simulink model "EE463_SoftwareProject2_q2_DCMotorDrive"  (R2017b)
settings: Solver=VariableStepDiscrete  StartTime=0.0  StopTime=2  RelTol=1e-3
libraries: powerlib x10
settings Model: Creator=mertelmas  LastModifiedBy=SiF

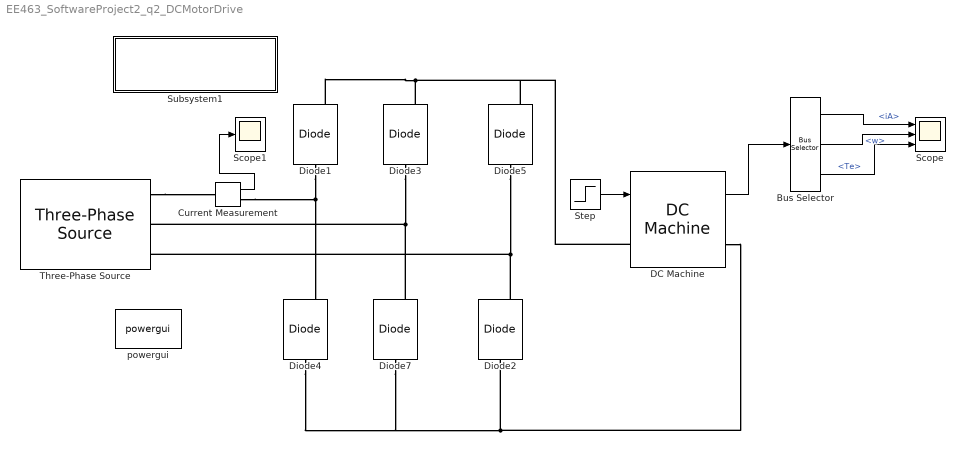
== system EE463_SoftwareProject2_q2_DCMotorDrive ==
  Bus Selector : BusSelector  OutputSignals=iA,w,Te
  Current Measurement : powerlib/Measurements/Current Measurement  PhasorSimulation=off  OutputType=Complex  PSBequivalent=0
  DC Machine : powerlib/Machines/DC Machine  PresetModel=No  MechanicalLoad=Torque TL  FieldType=Permanent magnet  ShowDetailedParameters=on  MeasurementBus=on  RLa="[ 10  0.01]"  RLf="[ 240  120]"  Laf=1.8  MachineConstant=Back-emf constant (V/rpm)  Ke=0.3  Kt=1.8  J=0.4  Bm=0  Tf=0  w0=0  Ifinit=0  TsPowergui=0  TsBlock=-1
  Diode{1..5,7} (6 alike) : powerlib/Power Electronics/Diode  Ron=0.001  Lon=0  Vf=0.8  IC=0  UseSnubber=0  Rs=500  Cs=250e-9  Measurements=on
  Scope : Scope  NumInputPorts=3
  Scope1 : Scope
  Step : Step  Time=0.000001  After=24  SampleTime=0
  Subsystem1 : Subsystem
      settings: OpenFcn=open_system('power_new_palette')
      mask Display: disp(sprintf('Open Simscape Power Systems\n(Specialized Technology)\nPalette Library'));
  Three-Phase Source : powerlib/Electrical Sources/Three-Phase Source  InternalConnection=Yg  VoltagePhases=off  Voltage=400  PhaseAngle=0  Voltage_phases=[25e3 25e3 25e3]/sqrt(3)  PhaseAngles_phases=[0 -120 +120]  Frequency=50  NonIdealSource=on  SpecifyImpedance=off  Resistance=100e-3  Inductance=100e-6  ShortCircuitLevel=100e6  BaseVoltage=25e3  XRratio=7  BusType=swing  Pref=10e3  Qref=0  Prefabc=[10e3, 10e3, 10e3]  Qrefabc=[0, 0, 0]  Qmin=-inf  Qmax=inf
  powergui : powerlib/powergui  Priority=1  SimulationMode=Discrete  SampleTime=1e-06  frequency=60  Iterations=50  frequencyindice=50  Pbase=100e6  ErrMax=1e-4  UnitsV=kV  UnitsW=MW  buscounter=0  FunctionMessages=off  echomessages=off  EnableUseOfTLC=off  CurrentSourceSwitches=off  DisableSnubberDevices=off  DisableRonSwitches=off  DisableVfSwitches=off  DisplayEquations=off  SolverType=Tustin/Backward Euler (TBE)  Interpol=off  ExternalGateDelay=off  methode=off  Ts=100  x0status=blocks  SPID=off  SwTol=0  HookPort=off  RestoreLinks=warning  ResistiveCurrentMeasurement=off  Frange=[0:2:500]  Ylog=off  Xlog=on  ShowGrid=off  save=off  variable=ZData  structure=ScopeData1  ZoomFFT=off  StartTime=1.6  cycles=15  DisplayStyle=1  fundamental=50  FreqAxis=off  MaxFrequency=1000  frequencyindicesteady=1  RmsSteady=1  display=off
  wires:
  Step/1 -> DC Machine/1
  DC Machine/1 -> Bus Selector/1
  Bus Selector/3 -> Scope/3  "<Te>"
  Bus Selector/1 -> Scope/1  "<iA>"
  Bus Selector/2 -> Scope/2  "<w>"
  Current Measurement/1 -> Scope1/1
  connections:
  Diode7/LConn1 -- Diode4/LConn1 -- DC Machine/RConn1 -- Diode2/LConn1
  Diode3/LConn1 -- Diode7/RConn1 -- Three-Phase Source/RConn2
  Diode2/RConn1 -- Diode5/LConn1 -- Three-Phase Source/RConn3
  Diode1/LConn1 -- Current Measurement/RConn1 -- Diode4/RConn1
  Diode1/RConn1 -- DC Machine/LConn1 -- Diode5/RConn1 -- Diode3/RConn1
  Three-Phase Source/RConn1 -- Current Measurement/LConn1

== system EE463_SoftwareProject2_q2_DCMotorDrive/Subsystem1 ==
